simulink model "HLS"  (R2021a)
settings: Solver=VariableStepAuto  StartTime=0.0  StopTime=33  RelTol=1e-3
undefined symbols (not defined in the file): A, N
libraries: hdlBasic x19, xbsIndex_r4 x1, JTAGRuntimeCosim_r4 x1
settings Model: Creator=sl186  LastModifiedBy=sl186

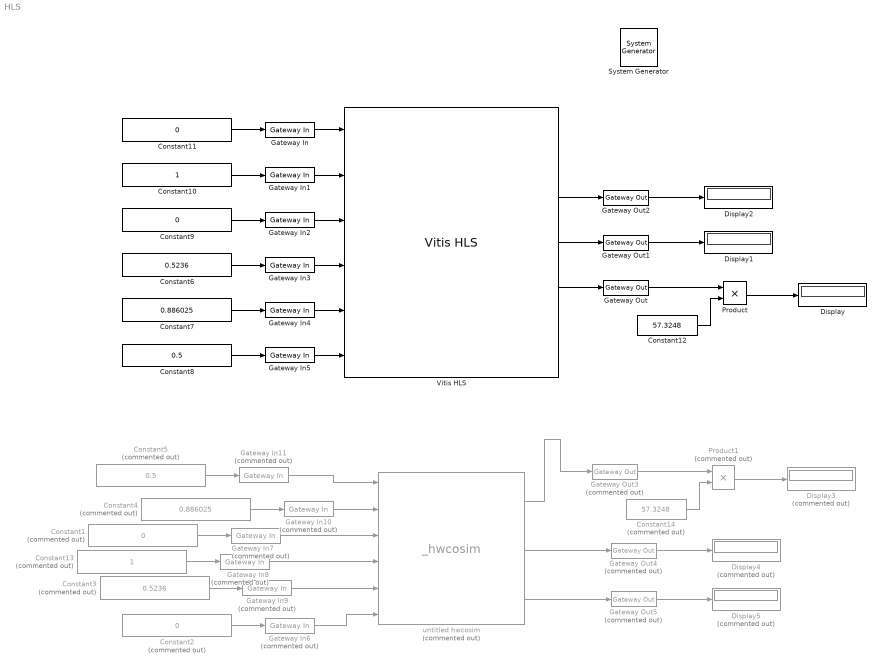
== system HLS ==
  " System Generator" : xbsIndex_r4/ System Generator  Tag=genX  xilinxfamily=zynq  part=xc7z020  speed=-1  package=clg484  synthesis_tool=Vivado  clock_wrapper=Clock Enables  directory=./netlist  proj_type=Vivado  Synth_file=Vivado Synthesis Defaults  Impl_file=Vivado Implementation Defaults  testbench=off  simulink_period=1  sysclk_period=10  dcm_input_clock_period=10  incr_netlist=off  trim_vbits=Everywhere in SubSystem  dbl_ovrd=According to Block Masks  core_generation=According to Block Masks  run_coregen=off  deprecated_control=off  eval_field=0  block_type=sysgen
  Constant1 : Constant  Commented=on  Value=0
  Constant10 : Constant
  Constant11 : Constant  Value=0
  Constant12 : Constant  Value=57.3248
  Constant13 : Constant  Commented=on
  Constant14 : Constant  Commented=on  Value=57.3248
  Constant2 : Constant  Commented=on  Value=0
  Constant3 : Constant  Commented=on  Value=0.5236
  Constant4 : Constant  Commented=on  Value=0.886025
  Constant5 : Constant  Commented=on  Value=0.5
  Constant6 : Constant  Value=0.5236
  Constant7 : Constant  Value=0.886025
  Constant8 : Constant  Value=0.5
  Constant9 : Constant  Value=0
  Display : Display
  Display1 : Display
  Display2 : Display
  Display3 : Display  Commented=on
  Display4 : Display  Commented=on
  Display5 : Display  Commented=on
  Gateway In : hdlBasic/Gateway In  gui_display_data_type=Boolean  arith_type=Boolean  n_bits=16  bin_pt=14  preci_type=Single  exp_width=8  frac_width=24  rows=1  columns=1  quantization="Round  (unbiased: +/- Inf)"  overflow=Saturate  period=1  UseAsADC=off  ADCChannel='1'  interface=None  automatic_assignment=on  address_offset=hex2dec('00')  intf_name=''  intf_description=''  default_value=0  timing_constraint=None  locs_specified=off  LOCs={}  io_standard={}  inherit_from_input=off  hdl_port=on  XmcBlockStatus=1  maskContainerNames=group4  block_type=gatewayin  block_config=sysgen:gateway_in_config  block_width_w=590  block_height_w=620  block_width=640  block_height=850
  Gateway In1 : hdlBasic/Gateway In  gui_display_data_type=Boolean  arith_type=Boolean  n_bits=16  bin_pt=14  preci_type=Single  exp_width=8  frac_width=24  rows=1  columns=1  quantization="Round  (unbiased: +/- Inf)"  overflow=Saturate  period=1  UseAsADC=off  ADCChannel='1'  interface=None  automatic_assignment=on  address_offset=hex2dec('00')  intf_name=''  intf_description=''  default_value=0  timing_constraint=None  locs_specified=off  LOCs={}  io_standard={}  inherit_from_input=off  hdl_port=on  XmcBlockStatus=1  maskContainerNames=group4  block_type=gatewayin  block_config=sysgen:gateway_in_config  block_width_w=590  block_height_w=620  block_width=640  block_height=850
  Gateway In10 : hdlBasic/Gateway In  Commented=on  gui_display_data_type=Fixed-point  arith_type=Signed (2's comp)  n_bits=16  bin_pt=14  preci_type=Single  exp_width=8  frac_width=24  rows=1  columns=1  quantization="Round  (unbiased: +/- Inf)"  overflow=Saturate  period=1  UseAsADC=off  ADCChannel='1'  interface=None  automatic_assignment=on  address_offset=hex2dec('00')  intf_name=''  intf_description=''  default_value=0  timing_constraint=None  locs_specified=off  LOCs={}  io_standard={}  inherit_from_input=off  hdl_port=on  XmcBlockStatus=1  maskContainerNames=group4  block_type=gatewayin  block_config=sysgen:gateway_in_config  block_width_w=590  block_height_w=620  block_width=640  block_height=850
  Gateway In11 : hdlBasic/Gateway In  Commented=on  gui_display_data_type=Fixed-point  arith_type=Signed (2's comp)  n_bits=16  bin_pt=14  preci_type=Single  exp_width=8  frac_width=24  rows=1  columns=1  quantization="Round  (unbiased: +/- Inf)"  overflow=Saturate  period=1  UseAsADC=off  ADCChannel='1'  interface=None  automatic_assignment=on  address_offset=hex2dec('00')  intf_name=''  intf_description=''  default_value=0  timing_constraint=None  locs_specified=off  LOCs={}  io_standard={}  inherit_from_input=off  hdl_port=on  XmcBlockStatus=1  maskContainerNames=group4  block_type=gatewayin  block_config=sysgen:gateway_in_config  block_width_w=590  block_height_w=620  block_width=640  block_height=850
  Gateway In2 : hdlBasic/Gateway In  gui_display_data_type=Boolean  arith_type=Boolean  n_bits=16  bin_pt=14  preci_type=Single  exp_width=8  frac_width=24  rows=1  columns=1  quantization="Round  (unbiased: +/- Inf)"  overflow=Saturate  period=1  UseAsADC=off  ADCChannel='1'  interface=None  automatic_assignment=on  address_offset=hex2dec('00')  intf_name=''  intf_description=''  default_value=0  timing_constraint=None  locs_specified=off  LOCs={}  io_standard={}  inherit_from_input=off  hdl_port=on  XmcBlockStatus=1  maskContainerNames=group4  block_type=gatewayin  block_config=sysgen:gateway_in_config  block_width_w=590  block_height_w=620  block_width=640  block_height=850
  Gateway In3 : hdlBasic/Gateway In  gui_display_data_type=Fixed-point  arith_type=Signed (2's comp)  n_bits=16  bin_pt=14  preci_type=Single  exp_width=8  frac_width=24  rows=1  columns=1  quantization="Round  (unbiased: +/- Inf)"  overflow=Saturate  period=1  UseAsADC=off  ADCChannel='1'  interface=None  automatic_assignment=on  address_offset=hex2dec('00')  intf_name=''  intf_description=''  default_value=0  timing_constraint=None  locs_specified=off  LOCs={}  io_standard={}  inherit_from_input=off  hdl_port=on  XmcBlockStatus=1  maskContainerNames=group4  block_type=gatewayin  block_config=sysgen:gateway_in_config  block_width_w=590  block_height_w=620  block_width=640  block_height=850
  Gateway In4 : hdlBasic/Gateway In  gui_display_data_type=Fixed-point  arith_type=Signed (2's comp)  n_bits=16  bin_pt=14  preci_type=Single  exp_width=8  frac_width=24  rows=1  columns=1  quantization="Round  (unbiased: +/- Inf)"  overflow=Saturate  period=1  UseAsADC=off  ADCChannel='1'  interface=None  automatic_assignment=on  address_offset=hex2dec('00')  intf_name=''  intf_description=''  default_value=0  timing_constraint=None  locs_specified=off  LOCs={}  io_standard={}  inherit_from_input=off  hdl_port=on  XmcBlockStatus=1  maskContainerNames=group4  block_type=gatewayin  block_config=sysgen:gateway_in_config  block_width_w=590  block_height_w=620  block_width=640  block_height=850
  Gateway In5 : hdlBasic/Gateway In  gui_display_data_type=Fixed-point  arith_type=Signed (2's comp)  n_bits=16  bin_pt=14  preci_type=Single  exp_width=8  frac_width=24  rows=1  columns=1  quantization="Round  (unbiased: +/- Inf)"  overflow=Saturate  period=1  UseAsADC=off  ADCChannel='1'  interface=None  automatic_assignment=on  address_offset=hex2dec('00')  intf_name=''  intf_description=''  default_value=0  timing_constraint=None  locs_specified=off  LOCs={}  io_standard={}  inherit_from_input=off  hdl_port=on  XmcBlockStatus=1  maskContainerNames=group4  block_type=gatewayin  block_config=sysgen:gateway_in_config  block_width_w=590  block_height_w=620  block_width=640  block_height=850
  Gateway In6 : hdlBasic/Gateway In  Commented=on  gui_display_data_type=Boolean  arith_type=Boolean  n_bits=16  bin_pt=14  preci_type=Single  exp_width=8  frac_width=24  rows=1  columns=1  quantization="Round  (unbiased: +/- Inf)"  overflow=Saturate  period=1  UseAsADC=off  ADCChannel='1'  interface=None  automatic_assignment=on  address_offset=hex2dec('00')  intf_name=''  intf_description=''  default_value=0  timing_constraint=None  locs_specified=off  LOCs={}  io_standard={}  inherit_from_input=off  hdl_port=on  XmcBlockStatus=1  maskContainerNames=group4  block_type=gatewayin  block_config=sysgen:gateway_in_config  block_width_w=590  block_height_w=620  block_width=640  block_height=850
  Gateway In7 : hdlBasic/Gateway In  Commented=on  gui_display_data_type=Boolean  arith_type=Boolean  n_bits=16  bin_pt=14  preci_type=Single  exp_width=8  frac_width=24  rows=1  columns=1  quantization="Round  (unbiased: +/- Inf)"  overflow=Saturate  period=1  UseAsADC=off  ADCChannel='1'  interface=None  automatic_assignment=on  address_offset=hex2dec('00')  intf_name=''  intf_description=''  default_value=0  timing_constraint=None  locs_specified=off  LOCs={}  io_standard={}  inherit_from_input=off  hdl_port=on  XmcBlockStatus=1  maskContainerNames=group4  block_type=gatewayin  block_config=sysgen:gateway_in_config  block_width_w=590  block_height_w=620  block_width=640  block_height=850
  Gateway In8 : hdlBasic/Gateway In  Commented=on  gui_display_data_type=Boolean  arith_type=Boolean  n_bits=16  bin_pt=14  preci_type=Single  exp_width=8  frac_width=24  rows=1  columns=1  quantization="Round  (unbiased: +/- Inf)"  overflow=Saturate  period=1  UseAsADC=off  ADCChannel='1'  interface=None  automatic_assignment=on  address_offset=hex2dec('00')  intf_name=''  intf_description=''  default_value=0  timing_constraint=None  locs_specified=off  LOCs={}  io_standard={}  inherit_from_input=off  hdl_port=on  XmcBlockStatus=1  maskContainerNames=group4  block_type=gatewayin  block_config=sysgen:gateway_in_config  block_width_w=590  block_height_w=620  block_width=640  block_height=850
  Gateway In9 : hdlBasic/Gateway In  Commented=on  gui_display_data_type=Fixed-point  arith_type=Signed (2's comp)  n_bits=16  bin_pt=14  preci_type=Single  exp_width=8  frac_width=24  rows=1  columns=1  quantization="Round  (unbiased: +/- Inf)"  overflow=Saturate  period=1  UseAsADC=off  ADCChannel='1'  interface=None  automatic_assignment=on  address_offset=hex2dec('00')  intf_name=''  intf_description=''  default_value=0  timing_constraint=None  locs_specified=off  LOCs={}  io_standard={}  inherit_from_input=off  hdl_port=on  XmcBlockStatus=1  maskContainerNames=group4  block_type=gatewayin  block_config=sysgen:gateway_in_config  block_width_w=590  block_height_w=620  block_width=640  block_height=850
  Gateway Out : hdlBasic/Gateway Out  inherit_from_input=off  hdl_port=on  rows=1  columns=1  UseAsDAC=off  DACChannel='1'  interface=None  automatic_assignment=on  address_offset=hex2dec('00')  intf_name=''  intf_description=''  timing_constraint=None  locs_specified=off  LOCs={}  io_standard={}  XmcBlockStatus=1  maskContainerNames=group4  block_type=gatewayout  block_config=sysgen:gateway_out_config  block_width_w=590  block_height_w=620  block_width=620  block_height=750
  Gateway Out1 : hdlBasic/Gateway Out  inherit_from_input=off  hdl_port=on  rows=1  columns=1  UseAsDAC=off  DACChannel='1'  interface=None  automatic_assignment=on  address_offset=hex2dec('00')  intf_name=''  intf_description=''  timing_constraint=None  locs_specified=off  LOCs={}  io_standard={}  XmcBlockStatus=1  maskContainerNames=group4  block_type=gatewayout  block_config=sysgen:gateway_out_config  block_width_w=590  block_height_w=620  block_width=620  block_height=750
  Gateway Out2 : hdlBasic/Gateway Out  inherit_from_input=off  hdl_port=on  rows=1  columns=1  UseAsDAC=off  DACChannel='1'  interface=None  automatic_assignment=on  address_offset=hex2dec('00')  intf_name=''  intf_description=''  timing_constraint=None  locs_specified=off  LOCs={}  io_standard={}  XmcBlockStatus=1  maskContainerNames=group4  block_type=gatewayout  block_config=sysgen:gateway_out_config  block_width_w=590  block_height_w=620  block_width=620  block_height=750
  Gateway Out3 : hdlBasic/Gateway Out  Commented=on  inherit_from_input=off  hdl_port=on  rows=1  columns=1  UseAsDAC=off  DACChannel='1'  interface=None  automatic_assignment=on  address_offset=hex2dec('00')  intf_name=''  intf_description=''  timing_constraint=None  locs_specified=off  LOCs={}  io_standard={}  XmcBlockStatus=1  maskContainerNames=group4  block_type=gatewayout  block_config=sysgen:gateway_out_config  block_width_w=590  block_height_w=620  block_width=620  block_height=750
  Gateway Out4 : hdlBasic/Gateway Out  Commented=on  inherit_from_input=off  hdl_port=on  rows=1  columns=1  UseAsDAC=off  DACChannel='1'  interface=None  automatic_assignment=on  address_offset=hex2dec('00')  intf_name=''  intf_description=''  timing_constraint=None  locs_specified=off  LOCs={}  io_standard={}  XmcBlockStatus=1  maskContainerNames=group4  block_type=gatewayout  block_config=sysgen:gateway_out_config  block_width_w=590  block_height_w=620  block_width=620  block_height=750
  Gateway Out5 : hdlBasic/Gateway Out  Commented=on  inherit_from_input=off  hdl_port=on  rows=1  columns=1  UseAsDAC=off  DACChannel='1'  interface=None  automatic_assignment=on  address_offset=hex2dec('00')  intf_name=''  intf_description=''  timing_constraint=None  locs_specified=off  LOCs={}  io_standard={}  XmcBlockStatus=1  maskContainerNames=group4  block_type=gatewayout  block_config=sysgen:gateway_out_config  block_width_w=590  block_height_w=620  block_width=620  block_height=750
  Product : Product
  Product1 : Product  Commented=on
  Vitis HLS : hdlBasic/Vitis HLS  anytable='C:\ELEC522\sl186\Assignment4\HLS\A4HLS\solution1'  fast_sim=off  display_datatype=on  rate_propagation_method=Simulink system period  model_file_path=''  latency=1  block_type=vitis_hls
      settings: infoedit=This block allows including C,C++ and SystemC source files in System Generator for DSP designs.
  untitled hwcosim : JTAGRuntimeCosim_r4/_hwcosim  Commented=on  clkSrc=Single Stepped  hasCombinationalPath=on  bitfileName=netlist\untitled.bit  skipConfig=off  dispPartInfo=off  useZynqReconfigScript=on  cable=Auto Detect  speed=N/A  cablePort=N/A  cableLocation=Local  shareCable=off  xmp=[]  software_settings=[]  design_xtable=|  binDir=[]  engineDll=JTAGCosimEngine.dll  cableWaitTime=10  bscanPos=-1  IRLengths=[]  useWaitBox=1  hasBufgmux=on  Scheme=Cosim  useCmdProc=1  hasProc=0  useImpact=0  printLogFile=0  userChain=2  XmcBlockStatus=0  maskContainerNames=tabcontainer1  block_type=jtagcosim  block_config=Sysgen:hwcosim_block_config
      | {
      |     'clkWrapper' => 'untitled',
      |     'burstMode' => false,
      |     'burstFifoDepth' => '1024',
      |     'shared_memories' => {},
      |     'clocksGcd' => 1,
      |     'device' => {
      |       'family' => 'zynq',
      |       'part' => 'xc7z020',
      |       'package' => 'clg484',
      |       'speed' => '-1',
      |     },
      |     'ports' => {
      |       'gateway_in5' => {
      |         'direction' => 'in',
      |         'width' => 16,
      |         'name' => 'gateway_in5',
      |         'period' => 1,
      |         'icon_text' => 'Gateway In5',
      |         'type' => 'Fix_16_14',
      |         'arithmetic_type' => 'xlSigned',
      |         'dat_file' => 'untitled_gateway_in5.dat',
      |         'bin_pt' => 14,
      |         'addr_offset' => 0,
      |         'bd_port_index' => 0,
      |       },
      |       'gateway_in4' => {
      |         'direction' => 'in',
      |         'width' => 16,
      |         'name' => 'gateway_in4',
      |         'period' => 1,
      |         'icon_text' => 'Gateway In4',
      |         'type' => 'Fix_16_14',
      |         'arithmetic_type' => 'xlSigned',
      |         'dat_file' => 'untitled_gateway_in4.dat',
      |         'bin_pt' => 14,
      |         'addr_offset' => 4,
      |         'bd_port_index' => 1,
      |       },
      |       'gateway_in2' => {
      |         'direction' => 'in',
      |         'width' => 1,
      |         'name' => 'gateway_in2',
      |         'period' => 1,
      |         'icon_text' => 'Gateway In2',
      |         'type' => 'Bool',
      |         'arithmetic_type' => 'xlUnsigned',
      |         'dat_file' => 'untitled_gateway_in2.dat',
      |         'bin_pt' => 0,
      |         'addr_offset' => 8,
      |         'bd_port_index' => 2,
      |       },
      |       'gateway_in1' => {
      |         'direction' => 'in',
      |         'width' => 1,
      |         'name' => 'gateway_in1',
      |         'period' => 1,
      |         'icon_text' => 'Gateway In1',
      |         'type' => 'Bool',
      |         'arithmetic_type' => 'xlUnsigned',
      |         'dat_file' => 'untitled_gateway_in1.dat',
      |         'bin_pt' => 0,
      |         'addr_offset' => 12,
      |         'bd_port_index' => 3,
      |       },
      |       'gateway_in3' => {
      |         'direction' => 'in',
      |         'width' => 16,
      |         'name' => 'gateway_in3',
      |         'period' => 1,
      |         'icon_text' => 'Gateway In3',
      |         'type' => 'Fix_16_14',
      |         'arithmetic_type' => 'xlSigned',
      |         'dat_file' => 'untitled_gateway_in3.dat',
      |         'bin_pt' => 14,
      |         'addr_offset' => 16,
      |         'bd_port_index' => 4,
      |       },
      |       'gateway_in' => {
      |         'direction' => 'in',
      |         'width' => 1,
      |         'name' => 'gateway_in',
      |         'period' => 1,
      |         'icon_text' => 'Gateway In',
      |         'type' => 'Bool',
      |         'arithmetic_type' => 'xlUnsigned',
      |         'dat_file' => 'untitled_gateway_in.dat',
      |         'bin_pt' => 0,
      |         'addr_offset' => 20,
      |         'bd_port_index' => 5,
      |       },
      |       'gateway_out' => {
      |         'direction' => 'out',
      |         'width' => 16,
      |         'name' => 'gateway_out',
      |         'period' => 1,
      |         'icon_text' => 'Gateway Out',
      |         'type' => 'Fix_16_14',
      |         'arithmetic_type' => 'xlSigned',
      |         'dat_file' => 'untitled_gateway_out.dat',
      |         'bin_pt' => 14,
      |         'addr_offset' => 24,
      |         'bd_port_index' => 0,
      |       },
      |       'gateway_out1' => {
      |         'direction' => 'out',
      |         'width' => 16,
      |         'name' => 'gateway_out1',
      |         'period' => 1,
      |         'icon_text' => 'Gateway Out1',
      |         'type' => 'Fix_16_14',
      |         'arithmetic_type' => 'xlSigned',
      |         'dat_file' => 'untitled_gateway_out1.dat',
      |         'bin_pt' => 14,
      |         'addr_offset' => 28,
      |         'bd_port_index' => 1,
      |       },
      |       'gateway_out2' => {
      |         'direction' => 'out',
      |         'width' => 16,
      |         'name' => 'gateway_out2',
      |         'period' => 1,
      |         'icon_text' => 'Gateway Out2',
      |         'type' => 'Fix_16_14',
      |         'arithmetic_type' => 'xlSigned',
      |         'dat_file' => 'untitled_gateway_out2.dat',
      |         'bin_pt' => 14,
      |         'addr_offset' => 32,
      |         'bd_port_index' => 2,
      |       },
      |     },
      |   }
  wires:
  Gateway In/1 -> Vitis HLS/1
  Gateway In1/1 -> Vitis HLS/2
  Gateway In2/1 -> Vitis HLS/3
  Gateway In3/1 -> Vitis HLS/4
  Gateway In4/1 -> Vitis HLS/5
  Gateway In5/1 -> Vitis HLS/6
  Vitis HLS/8 -> Gateway Out/1
  Gateway Out1/1 -> Display1/1
  Vitis HLS/6 -> Gateway Out1/1
  Gateway Out2/1 -> Display2/1
  Vitis HLS/4 -> Gateway Out2/1
  Constant11/1 -> Gateway In/1
  Constant10/1 -> Gateway In1/1
  Constant9/1 -> Gateway In2/1
  Constant6/1 -> Gateway In3/1
  Constant7/1 -> Gateway In4/1
  Constant8/1 -> Gateway In5/1
  Gateway Out/1 -> Product/1
  Constant12/1 -> Product/2
  Product/1 -> Display/1
  Constant5/1 -> Gateway In11/1
  Constant13/1 -> Gateway In8/1
  Constant4/1 -> Gateway In10/1
  Constant1/1 -> Gateway In7/1
  Constant3/1 -> Gateway In9/1
  Constant2/1 -> Gateway In6/1
  Gateway In6/1 -> untitled hwcosim/6
  Gateway In7/1 -> untitled hwcosim/3
  Gateway In8/1 -> untitled hwcosim/4
  Gateway In9/1 -> untitled hwcosim/5
  Gateway In10/1 -> untitled hwcosim/2
  Gateway In11/1 -> untitled hwcosim/1
  Constant14/1 -> Product1/2
  Product1/1 -> Display3/1
  Gateway Out3/1 -> Product1/1
  Gateway Out5/1 -> Display5/1
  Gateway Out4/1 -> Display4/1
  untitled hwcosim/3 -> Gateway Out5/1
  untitled hwcosim/2 -> Gateway Out4/1
  untitled hwcosim/1 -> Gateway Out3/1
